simulink model "SSpMon_Co"  (R2016b)
settings: configuration reference "CodeGenConfigSet" (kept outside this file)
values from neighbouring files (symbols this model uses):
  SSpMon_tiSRCMaxSply1DefDeb_C = Calibration.Parameter    [init_SSpMon_Co.m]
  SSpMon_tiSRCMaxSply1OKDeb_C = Calibration.Parameter    [init_SSpMon_Co.m]
  SSpMon_tiSRCMaxSplyDefDeb_C = Calibration.Parameter    [init_SSpMon_Co.m]
  SSpMon_tiSRCMaxSplyOKDeb_C = Calibration.Parameter    [init_SSpMon_Co.m]
  SSpMon_tiSRCMinSply1DefDeb_C = Calibration.Parameter    [init_SSpMon_Co.m]
  SSpMon_tiSRCMinSply1OKDeb_C = Calibration.Parameter    [init_SSpMon_Co.m]
  SSpMon_tiSRCMinSplyDefDeb_C = Calibration.Parameter    [init_SSpMon_Co.m]
  SSpMon_tiSRCMinSplyOKDeb_C = Calibration.Parameter    [init_SSpMon_Co.m]
  SSpMon_uSply1OutMax_C = Calibration.Parameter    [init_SSpMon_Co.m]
  SSpMon_uSply1OutMin_C = Calibration.Parameter    [init_SSpMon_Co.m]
  SSpMon_uSplyOutMax_C = Calibration.Parameter    [init_SSpMon_Co.m]
  SSpMon_uSplyOutMin_C = Calibration.Parameter    [init_SSpMon_Co.m]
undefined symbols (not defined in the file or in its folder): SSpMon_Co_DT
libraries: CXLib x12
settings Model: Creator=Administrator  LastModifiedBy=Administrator
settings ConfigSetRef: SourceLocation=Base Workspace

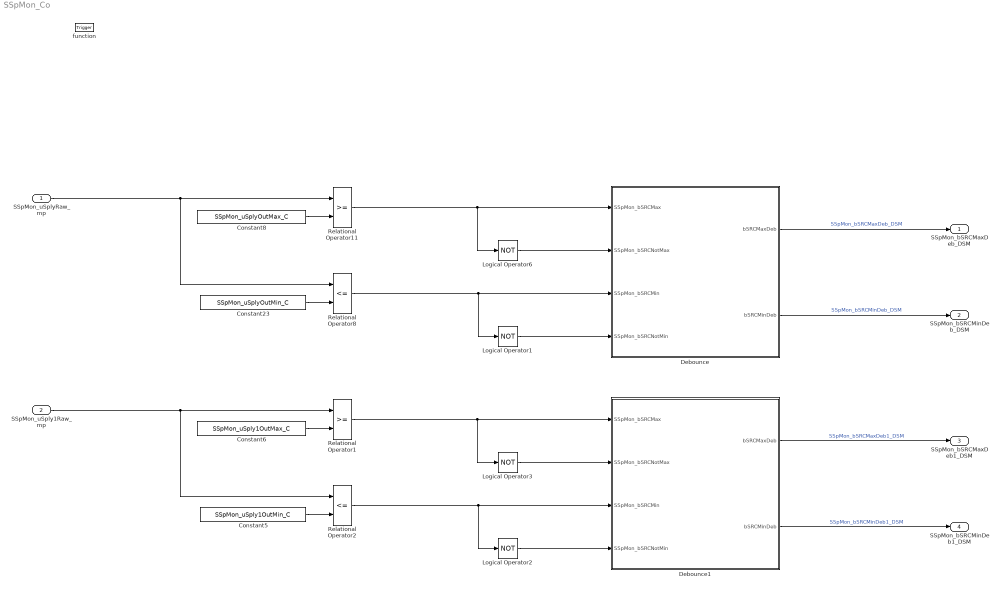
== system SSpMon_Co ==
  SSpMon_uSplyRaw_mp : Inport  Tag=mv  Description=Raw value of 12V sensor supply  OutMin=0  OutMax=5000  OutDataTypeStr=Ad_mv
  SSpMon_uSply1Raw_mp : Inport  Tag=mv  Description=Raw value of 12V sensor supply 1  Port=2  OutMin=0  OutMax=5000  OutDataTypeStr=Ad_mv
  function : TriggerPort  TriggerType=function-call  VariantControl=Variant
  Constant23 : Constant  Value=SSpMon_uSplyOutMin_C
  Constant5 : Constant  Value=SSpMon_uSply1OutMin_C
  Constant6 : Constant  Value=SSpMon_uSply1OutMax_C
  Constant8 : Constant  Value=SSpMon_uSplyOutMax_C
  Debounce : Subsystem
  Debounce1 : Subsystem
  Logical Operator{1..3,6} (4 alike) : Logic  Operator=NOT  AllPortsSameDT=off  OutDataTypeStr=boolean
  Relational Operator1 : RelationalOperator  OutDataTypeStr=boolean  RndMeth=Nearest  InputSameDT=on
  Relational Operator11 : RelationalOperator  OutDataTypeStr=boolean  RndMeth=Nearest  InputSameDT=on
  Relational Operator2 : RelationalOperator  Operator=<=  OutDataTypeStr=boolean  RndMeth=Nearest  InputSameDT=on
  Relational Operator8 : RelationalOperator  Operator=<=  OutDataTypeStr=boolean  RndMeth=Nearest  InputSameDT=on
  SSpMon_bSRCMaxDeb_DSM : Outport  Description=Status of SSpMon maximum signal range  OutMin=0  OutMax=1  OutDataTypeStr=boolean
  SSpMon_bSRCMinDeb_DSM : Outport  Description=Status of SSpMon minimum signal range  Port=2  OutMin=0  OutMax=1  OutDataTypeStr=boolean
  SSpMon_bSRCMaxDeb1_DSM : Outport  Description=Status of SSpMon1 maximum signal range  Port=3  OutMin=0  OutMax=1  OutDataTypeStr=boolean
  SSpMon_bSRCMinDeb1_DSM : Outport  Description=Status of SSpMon1 minimum signal range  Port=4  OutMin=0  OutMax=1  OutDataTypeStr=boolean
  wires:
  SSpMon_uSplyRaw_mp/1 -> Relational Operator8/1, Relational Operator11/1
  Constant8/1 -> Relational Operator11/2
  Constant23/1 -> Relational Operator8/2
  Relational Operator11/1 -> Logical Operator6/1, Debounce/1(SSpMon_bSRCMax)
  Relational Operator8/1 -> Logical Operator1/1, Debounce/3(SSpMon_bSRCMin)
  Debounce/1(bSRCMaxDeb) -> SSpMon_bSRCMaxDeb_DSM/1  "SSpMon_bSRCMaxDeb_DSM"
  Logical Operator6/1 -> Debounce/2(SSpMon_bSRCNotMax)
  Logical Operator1/1 -> Debounce/4(SSpMon_bSRCNotMin)
  Debounce/2(bSRCMinDeb) -> SSpMon_bSRCMinDeb_DSM/1  "SSpMon_bSRCMinDeb_DSM"
  SSpMon_uSply1Raw_mp/1 -> Relational Operator2/1, Relational Operator1/1
  Constant6/1 -> Relational Operator1/2
  Constant5/1 -> Relational Operator2/2
  Relational Operator1/1 -> Logical Operator3/1, Debounce1/1(SSpMon_bSRCMax)
  Relational Operator2/1 -> Logical Operator2/1, Debounce1/3(SSpMon_bSRCMin)
  Debounce1/1(bSRCMaxDeb) -> SSpMon_bSRCMaxDeb1_DSM/1  "SSpMon_bSRCMaxDeb1_DSM"
  Logical Operator3/1 -> Debounce1/2(SSpMon_bSRCNotMax)
  Logical Operator2/1 -> Debounce1/4(SSpMon_bSRCNotMin)
  Debounce1/2(bSRCMinDeb) -> SSpMon_bSRCMinDeb1_DSM/1  "SSpMon_bSRCMinDeb1_DSM"

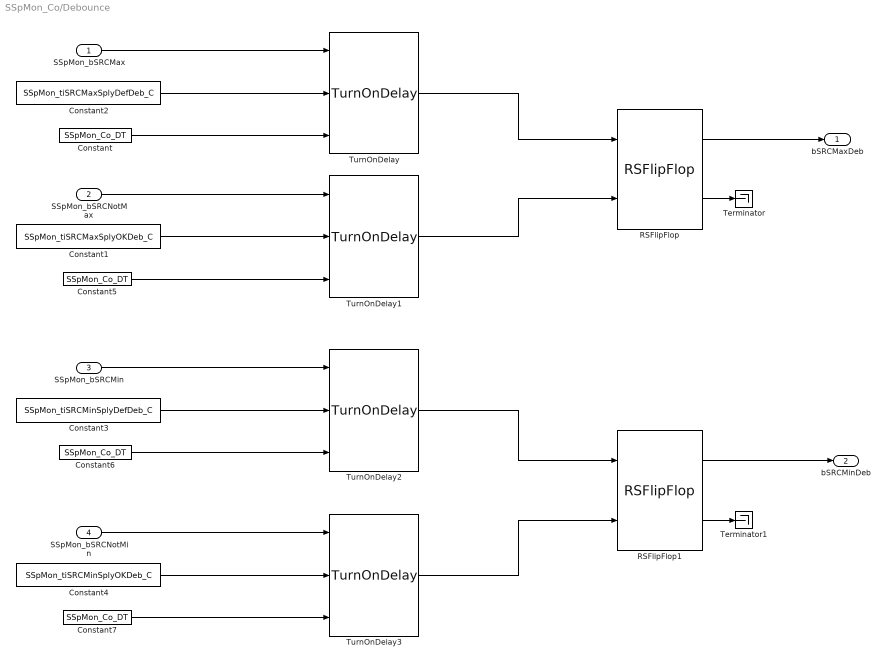
== system SSpMon_Co/Debounce ==
  SSpMon_bSRCMax : Inport
  SSpMon_bSRCNotMax : Inport  Port=2
  SSpMon_bSRCMin : Inport  Port=3
  SSpMon_bSRCNotMin : Inport  Port=4
  Constant{,5..7} (4 alike) : Constant  Value=SSpMon_Co_DT  OutDataTypeStr=Inherit: Inherit via back propagation
  Constant1 : Constant  Value=SSpMon_tiSRCMaxSplyOKDeb_C
  Constant2 : Constant  Value=SSpMon_tiSRCMaxSplyDefDeb_C
  Constant3 : Constant  Value=SSpMon_tiSRCMinSplyDefDeb_C
  Constant4 : Constant  Value=SSpMon_tiSRCMinSplyOKDeb_C
  RSFlipFlop : CXLib/RSFlipFlop
  RSFlipFlop1 : CXLib/RSFlipFlop
  Terminator : Terminator
  Terminator1 : Terminator
  TurnOnDelay{,1..3} (4 alike) : CXLib/TurnOnDelay
  bSRCMaxDeb : Outport
  bSRCMinDeb : Outport  Port=2
  wires:
  Constant7/1 -> TurnOnDelay3/3
  Constant6/1 -> TurnOnDelay2/3
  Constant5/1 -> TurnOnDelay1/3
  Constant/1 -> TurnOnDelay/3
  SSpMon_bSRCMax/1 -> TurnOnDelay/1
  RSFlipFlop1/2 -> Terminator1/1
  RSFlipFlop/2 -> Terminator/1
  Constant4/1 -> TurnOnDelay3/2
  TurnOnDelay3/1 -> RSFlipFlop1/2
  SSpMon_bSRCNotMin/1 -> TurnOnDelay3/1
  TurnOnDelay2/1 -> RSFlipFlop1/1
  SSpMon_bSRCMin/1 -> TurnOnDelay2/1
  SSpMon_bSRCNotMax/1 -> TurnOnDelay1/1
  TurnOnDelay/1 -> RSFlipFlop/1
  Constant2/1 -> TurnOnDelay/2
  Constant1/1 -> TurnOnDelay1/2
  Constant3/1 -> TurnOnDelay2/2
  TurnOnDelay1/1 -> RSFlipFlop/2
  RSFlipFlop/1 -> bSRCMaxDeb/1
  RSFlipFlop1/1 -> bSRCMinDeb/1

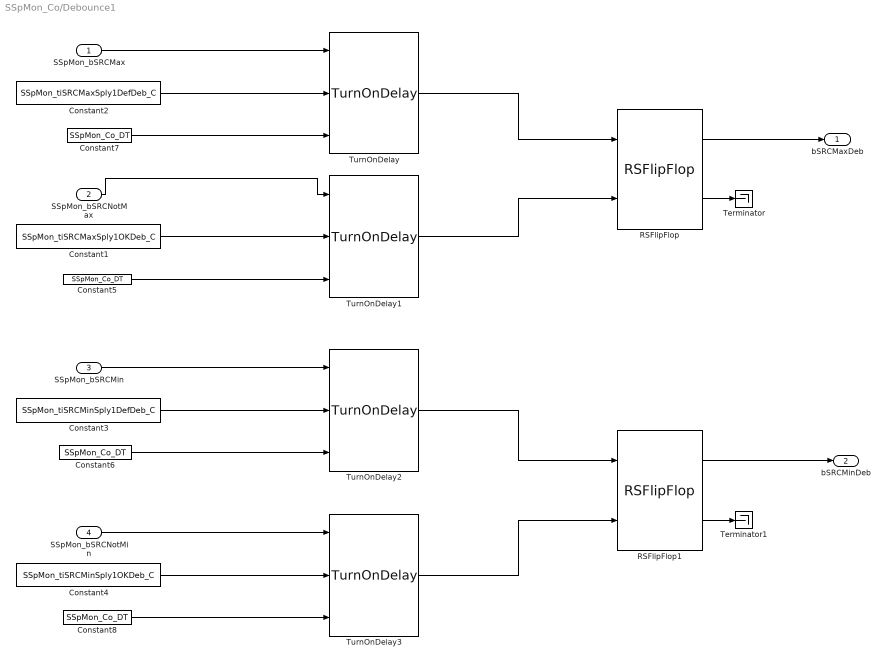
== system SSpMon_Co/Debounce1 ==
  SSpMon_bSRCMax : Inport
  SSpMon_bSRCNotMax : Inport  Port=2
  SSpMon_bSRCMin : Inport  Port=3
  SSpMon_bSRCNotMin : Inport  Port=4
  Constant1 : Constant  Value=SSpMon_tiSRCMaxSply1OKDeb_C
  Constant2 : Constant  Value=SSpMon_tiSRCMaxSply1DefDeb_C
  Constant3 : Constant  Value=SSpMon_tiSRCMinSply1DefDeb_C
  Constant4 : Constant  Value=SSpMon_tiSRCMinSply1OKDeb_C
  Constant{5..8} (4 alike) : Constant  Value=SSpMon_Co_DT  OutDataTypeStr=Inherit: Inherit via back propagation
  RSFlipFlop : CXLib/RSFlipFlop
  RSFlipFlop1 : CXLib/RSFlipFlop
  Terminator : Terminator
  Terminator1 : Terminator
  TurnOnDelay{,1..3} (4 alike) : CXLib/TurnOnDelay
  bSRCMaxDeb : Outport
  bSRCMinDeb : Outport  Port=2
  wires:
  Constant8/1 -> TurnOnDelay3/3
  Constant6/1 -> TurnOnDelay2/3
  Constant5/1 -> TurnOnDelay1/3
  Constant7/1 -> TurnOnDelay/3
  SSpMon_bSRCMax/1 -> TurnOnDelay/1
  RSFlipFlop1/2 -> Terminator1/1
  RSFlipFlop/2 -> Terminator/1
  Constant4/1 -> TurnOnDelay3/2
  TurnOnDelay3/1 -> RSFlipFlop1/2
  SSpMon_bSRCNotMin/1 -> TurnOnDelay3/1
  TurnOnDelay2/1 -> RSFlipFlop1/1
  SSpMon_bSRCMin/1 -> TurnOnDelay2/1
  SSpMon_bSRCNotMax/1 -> TurnOnDelay1/1
  TurnOnDelay/1 -> RSFlipFlop/1
  Constant2/1 -> TurnOnDelay/2
  Constant1/1 -> TurnOnDelay1/2
  Constant3/1 -> TurnOnDelay2/2
  TurnOnDelay1/1 -> RSFlipFlop/2
  RSFlipFlop/1 -> bSRCMaxDeb/1
  RSFlipFlop1/1 -> bSRCMinDeb/1
